simulink model "TestModel_CreatePort"  (R2025b)
settings: Solver=VariableStepAuto  StartTime=0.0  StopTime=10.0  RelTol=1e-3
settings Model: Creator=Administrator  LastModifiedBy=Administrator

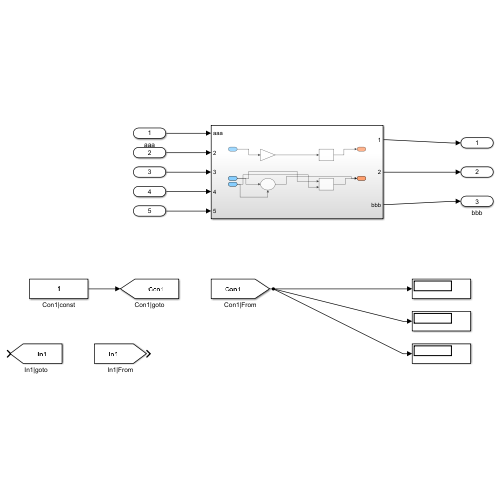
[thumbnail: Simulink's stored preview of the top-level diagram]
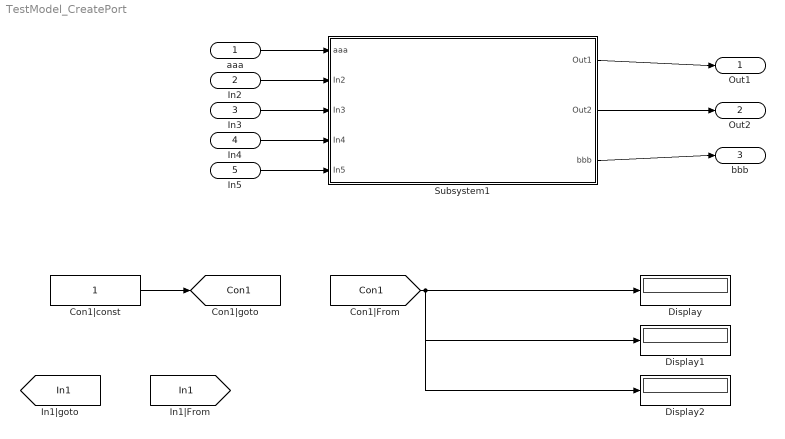
== system TestModel_CreatePort ==
  aaa : Inport
  In2 : Inport  Port=2
  In3 : Inport  Port=3
  In4 : Inport  Port=4
  In5 : Inport  Port=5
  Con1|const : Constant
  Display : Display
  Display1 : Display
  Display2 : Display
  Subsystem1 : Subsystem
  Out1 : Outport
  Out2 : Outport  Port=2
  bbb : Outport  Port=3
  tag scope: Con1=global, In1=global
  wires:
  Con1|const/1 -> [Con1]
  [Con1] -> Display2/1, Display1/1, Display/1
  Subsystem1/1(Out1) -> Out1/1
  Subsystem1/2(Out2) -> Out2/1
  Subsystem1/3(bbb) -> bbb/1
  aaa/1 -> Subsystem1/1(aaa)
  In2/1 -> Subsystem1/2(In2)
  In3/1 -> Subsystem1/3(In3)
  In4/1 -> Subsystem1/4(In4)
  In5/1 -> Subsystem1/5(In5)

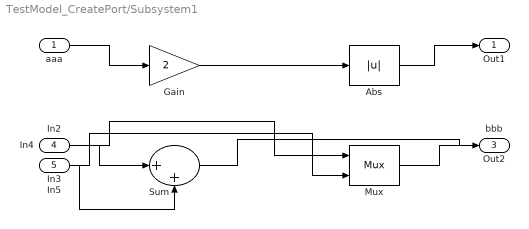
== system TestModel_CreatePort/Subsystem1 ==
  aaa : Inport
  In2 : Inport  Port=2
  In3 : Inport  Port=3
  In4 : Inport  Port=4
  In5 : Inport  Port=5
  Abs : Abs
  Gain : Gain  Gain=2
  Mux : Mux  Inputs=2
  Sum : Sum  Inputs=|++
  Out1 : Outport
  Out2 : Outport  Port=2
  bbb : Outport  Port=3
  wires:
  Gain/1 -> Abs/1
  aaa/1 -> Gain/1
  In2/1 -> Mux/1
  In3/1 -> Mux/2
  In4/1 -> Sum/1
  In5/1 -> Sum/2
  Abs/1 -> Out1/1
  Mux/1 -> Out2/1
  Sum/1 -> bbb/1
